simulink model "veryfirstmodel"  (R2016a)
settings: Solver=ode4  StartTime=0.0  StopTime=1  FixedStep=1e-3  RelTol=1e-3
settings Model: Creator=ugurm  LastModifiedBy=mesutto
settings DataIOCC: LimitDataPoints=on  SaveFormat=Array
settings DebuggingCC: UnderspecifiedInitializationDetection=Classic  MergeDetectMultiDrivingBlocksExec=none  SolverPrmCheckMsg=warning  StateNameClashWarn=warning
settings HardwareCC: ProdBitPerPointer=32  ProdLargestAtomicFloat=None  ProdIntDivRoundTo=Undefined  ProdEndianess=Unspecified  ProdWordSize=32  ProdHWDeviceType=32-bit Generic
settings ModelReferenceCC: PropagateSignalLabelsOutOfModel=off
settings ConfigComp: CovModelRefEnable=Off
settings ConfigurationSet: Description=SimMechanics 2G

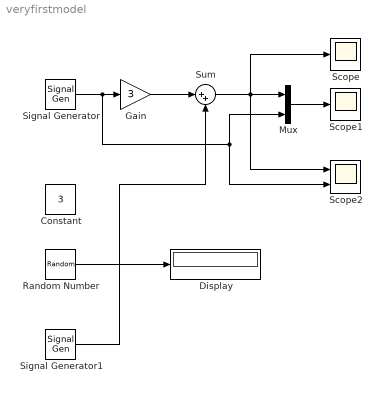
== system veryfirstmodel ==
  Constant : Constant  Value=3
  Display : Display
  Gain : Gain  Gain=3
  Mux : Mux  Inputs=2
  Random Number : RandomNumber  Variance=0.1  SampleTime=1e-2
  Scope : Scope
  Scope1 : Scope
  Scope2 : Scope  NumInputPorts=2
  Signal Generator : SignalGenerator  Frequency=50
  Signal Generator1 : SignalGenerator  Amplitude=0.4  Frequency=150
  Sum : Sum  Inputs=|++
  wires:
  Signal Generator/1 -> Mux/2, Scope2/2, Gain/1
  Gain/1 -> Sum/1
  Signal Generator1/1 -> Sum/2
  Sum/1 -> Scope2/1, Mux/1, Scope/1
  Mux/1 -> Scope1/1
  Random Number/1 -> Display/1
